simulink subsystem "HVAC_ECU"  (R2021a)
settings: Solver=VariableStepAuto  StartTime=0.0  StopTime=10.0  RelTol=1e-3
settings Model: Creator=prasad  LastModifiedBy=Sai229

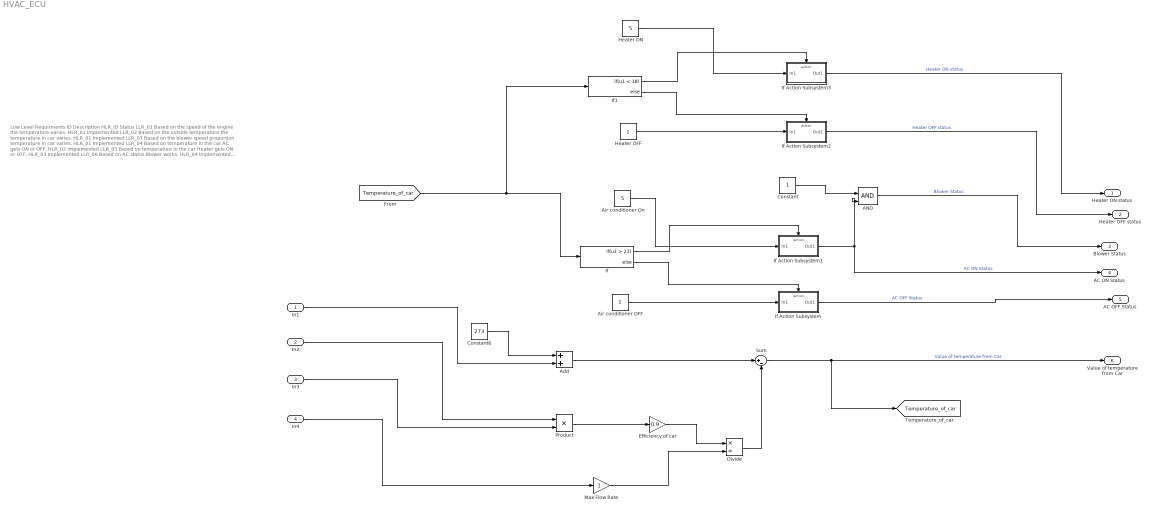
== system HVAC_ECU ==
  note: Low Level Requirments
      | ID
      | Description
      | HLR_ID
      | Status
      |
      | LLR_01
      | Based on the speed of the engine the temperature varies.
      | HLR_01
      | Implemented
      |
      | LLR_02
      | Based on the outside temperature the temperature in car varies.
      | HLR_01
      | Implemented
      |
      | LLR_03
      | Based on the blower speed proportion temperature in car varies.
      | HLR_01
      | Implemented
      |
      | LLR_04
      | Based on temperature in the car AC gets ON or OFF.
      | HLR_02
      | Implemented
      |
      | LLR_05
      | Based on temperature in the car Heater gets ON or OFF.
      | HLR_03
      | Implemented
      |
      | LLR_06
      | Based on AC status Blower works.
      | HLR_04
      | Implemented
      |
      | LOGIC:
      | STEP 1. Taking values of engine temperature and comp Torque and multipled and given to efficiency(gain).
      | STEP 2. Blower speed proportion and given toMaximum flow rate(gain).
      | STEP 3. Both values were given to divide block.
      | STEP 4. Internal Temperature is in degrees and after it converted into kelvin.
      | STEP 5. Subtract of both values, then the temperature will display on the Display block.
      | 1.Based on temperature the AC is getting on.
      | a.If the value(temperature) is greater than 23 then AC should be on.
      | b.Else the AC should be off.
      | 2. Based on AC status Blower Works.
      | 3. Based on temperature the Blower is getting on.
      | a.If the value(temperature) is less than 18 then Heater should be on.
      | b.Else the Heater should be off.
  In1 : Inport
  In2 : Inport  Port=2
  In3 : Inport  Port=3
  In4 : Inport  Port=4
  AND : Logic  IconShape=distinctive  AllPortsSameDT=off  OutDataTypeStr=boolean
  Add : Sum
  Air conditioner OFF : Constant
  Air conditioner On : Constant  Value=5
  Constant : Constant
  Constant6 : Constant  Value=273
  Divide : Product  Inputs=*/
  Efficiency of car : Gain  Gain=0.9
  Heater OFF : Constant
  Heater ON : Constant  Value=5
  If : If  IfExpression=u1 > 23
  If Action Subsystem : Subsystem  TreatAsAtomicUnit=on
  If Action Subsystem1 : Subsystem  TreatAsAtomicUnit=on
  If Action Subsystem2 : Subsystem  TreatAsAtomicUnit=on
  If Action Subsystem3 : Subsystem  TreatAsAtomicUnit=on
  If1 : If  IfExpression=u1 < 18
  Max Flow Rate : Gain
  Product : Product
  Sum : Sum  Inputs=|+-
  Heater ON status : Outport
  Heater OFF status : Outport  Port=2
  Blower Status : Outport  Port=3
  AC ON Status : Outport  Port=4
  AC OFF Status : Outport  Port=5
  Value of temperature from Car : Outport  Port=6
  tag scope: Temperature_of_car=global
  wires:
  Sum/1 -> [Temperature_of_car], Value of temperature from Car/1  "Value of temperature from Car"
  If Action Subsystem/1(Out1) -> AC OFF Status/1  "AC OFF Status"
  Divide/1 -> Sum/2
  [Temperature_of_car] -> If/1, If1/1
  If1/1 -> If Action Subsystem3/Action
  Constant/1 -> AND/1
  Efficiency of car/1 -> Divide/1
  If Action Subsystem3/1(Out1) -> Heater ON status/1  "Heater ON status"
  Air conditioner OFF/1 -> If Action Subsystem/1(In1)
  Max Flow Rate/1 -> Divide/2
  Add/1 -> Sum/1
  If1/2 -> If Action Subsystem2/Action
  Heater OFF/1 -> If Action Subsystem2/1(In1)
  If Action Subsystem1/1(Out1) -> AND/2, AC ON Status/1  "AC ON Status"
  Heater ON/1 -> If Action Subsystem3/1(In1)
  Constant6/1 -> Add/1
  In2/1 -> Product/1
  In3/1 -> Product/2
  In1/1 -> Add/2
  If/2 -> If Action Subsystem/Action
  Product/1 -> Efficiency of car/1
  In4/1 -> Max Flow Rate/1
  If Action Subsystem2/1(Out1) -> Heater OFF status/1  "Heater OFF status"
  AND/1 -> Blower Status/1  "Blower Status"
  If/1 -> If Action Subsystem1/Action
  Air conditioner On/1 -> If Action Subsystem1/1(In1)

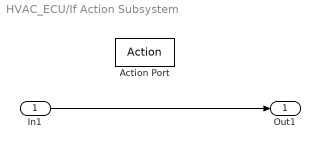
== system HVAC_ECU/If Action Subsystem ==
  In1 : Inport
  Action Port : ActionPort
  Out1 : Outport
  wires:
  In1/1 -> Out1/1

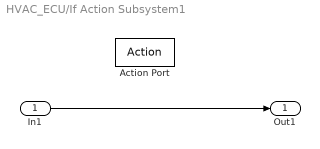
== system HVAC_ECU/If Action Subsystem1 ==
  In1 : Inport
  Action Port : ActionPort
  Out1 : Outport
  wires:
  In1/1 -> Out1/1

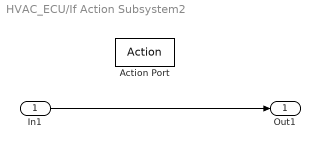
== system HVAC_ECU/If Action Subsystem2 ==
  In1 : Inport
  Action Port : ActionPort
  Out1 : Outport
  wires:
  In1/1 -> Out1/1

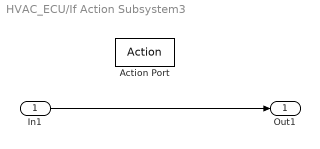
== system HVAC_ECU/If Action Subsystem3 ==
  In1 : Inport
  Action Port : ActionPort
  Out1 : Outport
  wires:
  In1/1 -> Out1/1
